simulink model "test2015b"  (R2015b)
settings: Solver=VariableStepAuto  StartTime=0.0  StopTime=10.0  RelTol=1e-3
settings Model: Creator=hjorl  LastModifiedBy=stefa
settings DataIOCC: LimitDataPoints=off
settings DebuggingCC: AllowSymbolicDim=on
settings ModelReferenceCC: PropagateSignalLabelsOutOfModel=on
settings GRTTargetCC: GeneratePreprocessorConditionals=Disable all
settings ConfigComp: CovModelRefEnable=Off

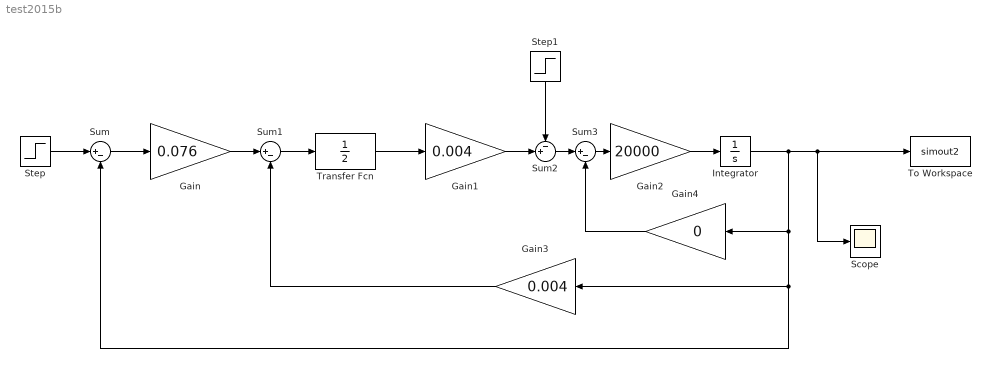
== system test2015b ==
  Gain : Gain  Gain=0.076
  Gain1 : Gain  Gain=0.004
  Gain2 : Gain  Gain=20000
  Gain3 : Gain  Gain=0.004
  Gain4 : Gain  Gain=0
  Integrator : Integrator
  Scope : Scope
  Step : Step  After=500  SampleTime=0
  Step1 : Step  Before=0.008  After=0.008  SampleTime=0
  Sum : Sum  Inputs=|+-
  Sum1 : Sum  Inputs=|+-
  Sum2 : Sum  Inputs=-+|
  Sum3 : Sum  Inputs=|+-
  To Workspace : ToWorkspace  VariableName=simout2  SaveFormat=Structure With Time  SampleTime=-1
  Transfer Fcn : TransferFcn  Denominator=[0 2]
  wires:
  Step/1 -> Sum/1
  Integrator/1 -> Gain4/1, Gain3/1, Sum/2, Scope/1, To Workspace/1
  Transfer Fcn/1 -> Gain1/1
  Sum/1 -> Gain/1
  Sum1/1 -> Transfer Fcn/1
  Gain/1 -> Sum1/1
  Gain1/1 -> Sum2/2
  Sum2/1 -> Sum3/1
  Sum3/1 -> Gain2/1
  Gain2/1 -> Integrator/1
  Gain4/1 -> Sum3/2
  Gain3/1 -> Sum1/2
  Step1/1 -> Sum2/1
